simulink model "String_Efficiency_Model_of_Suspension_Insulator"  (R2023b)
settings: Solver=VariableStepAuto  StartTime=0.0  StopTime=1.0  RelTol=1e-3
libraries: spsSeriesRLCBranchLib x8, spsRMSLib x4, spsVoltageMeasurementLib x4, spsGroundLib x2, spsACVoltageSourceLib x1, sps_lib x1
settings Model: Creator=HP  LastModifiedBy=HP

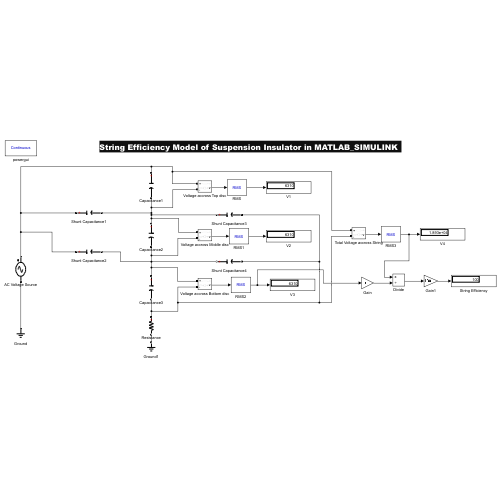
[thumbnail: Simulink's stored preview of the top-level diagram]
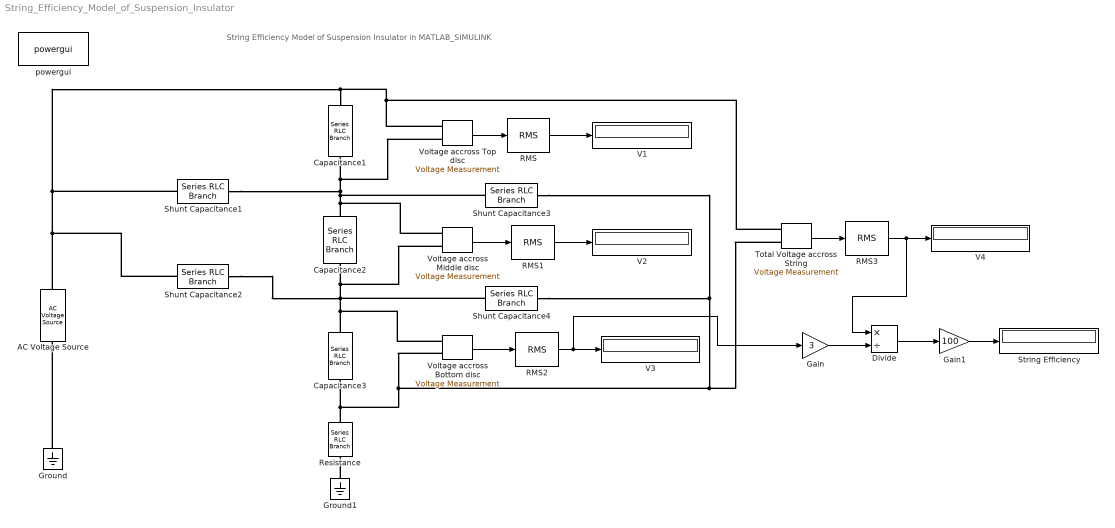
== system String_Efficiency_Model_of_Suspension_Insulator ==
  note: String Efficiency Model of Suspension Insulator in MATLAB_SIMULINK
  AC Voltage Source : spsACVoltageSourceLib/AC Voltage Source  Amplitude=1.414*19.05e3  Phase=0  Frequency=60  SampleTime=0  Measurements=None  BusType=swing  Pref=10e3  Qref=0  Qmin=-inf  Qmax=+inf
  Capacitance1 : spsSeriesRLCBranchLib/Series RLC Branch  LConnTagsString=__new0  RConnTagsString=__new0  BranchType=C  Resistance=1  Inductance=1e-3  SetiL0=off  InitialCurrent=0  Capacitance=1e-6  Setx0=off  InitialVoltage=0  Measurements=None
  Capacitance2 : spsSeriesRLCBranchLib/Series RLC Branch  LConnTagsString=__new0  RConnTagsString=__new0  BranchType=C  Resistance=1  Inductance=1e-3  SetiL0=off  InitialCurrent=0  Capacitance=1e-6  Setx0=off  InitialVoltage=0  Measurements=None
  Capacitance3 : spsSeriesRLCBranchLib/Series RLC Branch  LConnTagsString=__new0  RConnTagsString=__new0  BranchType=C  Resistance=1  Inductance=1e-3  SetiL0=off  InitialCurrent=0  Capacitance=1e-6  Setx0=off  InitialVoltage=0  Measurements=None
  Divide : Product  Inputs=*/
  Gain : Gain  Gain=3
  Gain1 : Gain  Gain=100
  Ground : spsGroundLib/Ground  LConnTagsString=a
  Ground1 : spsGroundLib/Ground  LConnTagsString=a
  RMS{,1..3} (4 alike) : spsRMSLib/RMS  TrueRMS=on  Freq=60  RMSInit=0  Ts=0
  Resistance : spsSeriesRLCBranchLib/Series RLC Branch  LConnTagsString=__new0  RConnTagsString=__new0  BranchType=R  Resistance=1  Inductance=1e-3  SetiL0=off  InitialCurrent=0  Capacitance=1e-6  Setx0=off  InitialVoltage=0  Measurements=None
  Shunt Capacitance1 : spsSeriesRLCBranchLib/Series RLC Branch  LConnTagsString=__new0  RConnTagsString=__new0  BranchType=C  Resistance=1  Inductance=1e-3  SetiL0=off  InitialCurrent=0  Capacitance=0.1e-6  Setx0=off  InitialVoltage=0  Measurements=None
  Shunt Capacitance2 : spsSeriesRLCBranchLib/Series RLC Branch  LConnTagsString=__new0  RConnTagsString=__new0  BranchType=C  Resistance=1  Inductance=1e-3  SetiL0=off  InitialCurrent=0  Capacitance=0.1e-6  Setx0=off  InitialVoltage=0  Measurements=None
  Shunt Capacitance3 : spsSeriesRLCBranchLib/Series RLC Branch  LConnTagsString=__new0  RConnTagsString=__new0  BranchType=C  Resistance=1  Inductance=1e-3  SetiL0=off  InitialCurrent=0  Capacitance=0.05e-6  Setx0=off  InitialVoltage=0  Measurements=None
  Shunt Capacitance4 : spsSeriesRLCBranchLib/Series RLC Branch  LConnTagsString=__new0  RConnTagsString=__new0  BranchType=C  Resistance=1  Inductance=1e-3  SetiL0=off  InitialCurrent=0  Capacitance=0.2e-6  Setx0=off  InitialVoltage=0  Measurements=None
  String Efficiency : Display
  Total Voltage accross String : spsVoltageMeasurementLib/Voltage Measurement  PhasorSimulation=off  OutputType=Complex  PSBequivalent=0
  V{1..4} (4 alike) : Display
  Voltage accross Bottom disc : spsVoltageMeasurementLib/Voltage Measurement  PhasorSimulation=off  OutputType=Complex  PSBequivalent=0
  Voltage accross Middle disc : spsVoltageMeasurementLib/Voltage Measurement  PhasorSimulation=off  OutputType=Complex  PSBequivalent=0
  Voltage accross Top disc : spsVoltageMeasurementLib/Voltage Measurement  PhasorSimulation=off  OutputType=Complex  PSBequivalent=0
  powergui : sps_lib/powergui  Priority=1  SimulationMode=Continuous  SampleTime=50e-6  frequency=60  Iterations=50  frequencyindice=60  Pbase=100e6  ErrMax=1e-4  UnitsV=kV  UnitsW=MW  buscounter=0  FunctionMessages=off  echomessages=off  EnableUseOfTLC=off  CurrentSourceSwitches=off  DisableSnubberDevices=off  DisableRonSwitches=off  DisableVfSwitches=off  DisplayEquations=off  AutomaticDiscreteSolvers=off  SolverType=Tustin/Backward Euler (TBE)  Interpol=off  ExternalGateDelay=off  methode=off  Ts=100  x0status=blocks  SPID=on  SwTol=0  HookPort=off  NonlinearTolerance=1e-4  nMaxIteration=100  ContinueOnMaxIteration=off  RestoreLinks=warning  ResistiveCurrentMeasurement=off  Frange=[0:2:500]  Ylog=off  Xlog=on  ShowGrid=off  save=off  variable=ZData  structure=0  ZoomFFT=off  StartTime=0.0  cycles=1  DisplayStyle=1  fundamental=60  FreqAxis=off  MaxFrequency=1000  frequencyindicesteady=1  RmsSteady=1  display=off
  wires:
  Voltage accross Top disc/1 -> RMS/1
  RMS/1 -> V1/1
  Voltage accross Middle disc/1 -> RMS1/1
  Voltage accross Bottom disc/1 -> RMS2/1
  RMS1/1 -> V2/1
  RMS2/1 -> Gain/1, V3/1
  Total Voltage accross String/1 -> RMS3/1
  RMS3/1 -> V4/1, Divide/1
  Gain/1 -> Divide/2
  Divide/1 -> Gain1/1
  Gain1/1 -> String Efficiency/1
  connections:
  Ground/LConn1 -- AC Voltage Source/LConn1
  Capacitance2/LConn1 -- Voltage accross Middle disc/LConn1 -- Shunt Capacitance1/RConn1 -- Voltage accross Top disc/LConn2 -- Capacitance1/RConn1 -- Shunt Capacitance3/LConn1
  Capacitance3/LConn1 -- Voltage accross Bottom disc/LConn1 -- Voltage accross Middle disc/LConn2 -- Capacitance2/RConn1 -- Shunt Capacitance4/LConn1 -- Shunt Capacitance2/RConn1
  AC Voltage Source/RConn1 -- Shunt Capacitance1/LConn1 -- Capacitance1/LConn1 -- Total Voltage accross String/LConn1 -- Voltage accross Top disc/LConn1 -- Shunt Capacitance2/LConn1
  Resistance/LConn1 -- Capacitance3/RConn1 -- Shunt Capacitance4/RConn1 -- Shunt Capacitance3/RConn1 -- Total Voltage accross String/LConn2 -- Voltage accross Bottom disc/LConn2
  Ground1/LConn1 -- Resistance/RConn1
